simulink model "swingup_LQR"  (R2020b)
settings: Solver=VariableStepAuto  StartTime=0.0  StopTime=40  RelTol=1e-3
values from neighbouring files (symbols this model uses):
  g = 9.81    [upright_LQR.m]
  h = 0.01    [upright_LQR.m]
  Jp = mp*Lp^2/3    (= 0.000133128)    [upright_LQR.m]
  K = lqr(A, B, q_lqr, r_lqr)    [upright_LQR.m]
  ke = 0.1    [upright_LQR.m]
  kt = 0.042    [upright_LQR.m]
  l = Lp/2    (= 0.0645)    [upright_LQR.m]
  mp = 0.024    [upright_LQR.m]
  mr = 0.095    [upright_LQR.m]
  r = 0.085    [upright_LQR.m]
  Rm = 8.4    [upright_LQR.m]
  u_max = 10    [upright_LQR.m]
undefined symbols (not defined in the file or in its folder): Humusoft, MF634
libraries: simulink_extras x4, simulink x4, sldrtlib x2, eeLuenbergerObserver x1
settings Model: Creator=zhehanli  LastModifiedBy=zhehanli

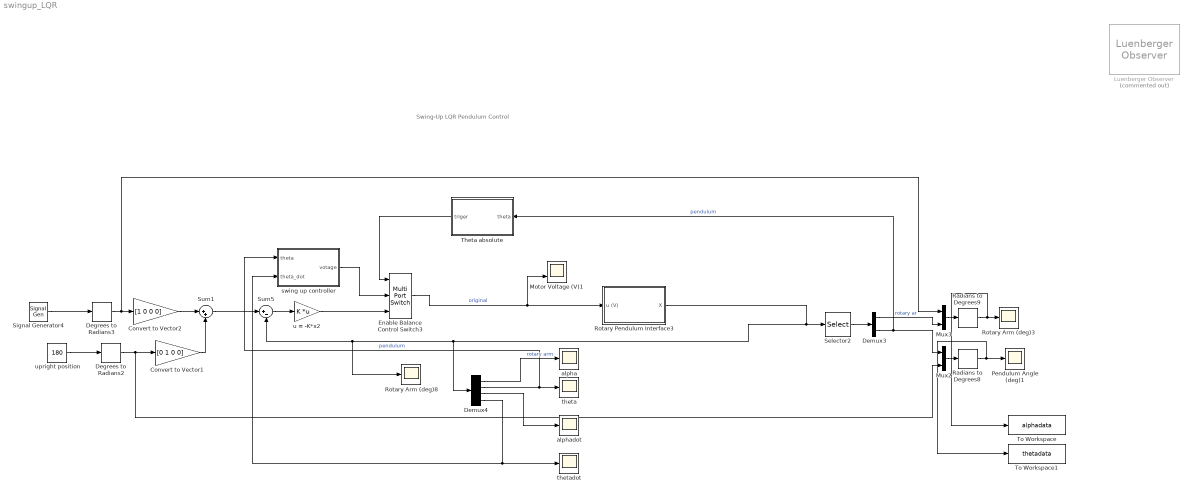
== system swingup_LQR ==
  note: Swing-Up LQR Pendulum Control
  Convert to Vector1 : Gain  Gain=[0 1 0 0]
  Convert to Vector2 : Gain  Gain=[1 0 0 0]
  Degrees to Radians2 : simulink_extras/Transformations/Degrees to Radians
  Degrees to Radians3 : simulink_extras/Transformations/Degrees to Radians
  Demux3 : Demux  Outputs=2
  Demux4 : Demux
  Enable Balance Control Switch3 : MultiPortSwitch  DataPortOrder=Zero-based contiguous  Inputs=2  zeroidx=on
  Luenberger Observer : eeLuenbergerObserver/Luenberger Observer  Commented=on  StateSpaceType=Discrete-time  Ad=1  Bd=1  Cd=1  Dd=1  A=1  B=1  C=1  D=1  ObserverDesign=Desired eigenvalues  Ld=1  DesiredEigenvalues=0  x0=0  Tsd=0.1  Ts=0.1
      settings: SourceProductBaseCode=PS
  Motor Voltage (V)1 : Scope  NumInputPorts=2
  Mux2 : Mux  Inputs=2
  Mux3 : Mux  Inputs=2
  Pendulum Angle (deg)1 : Scope
  Radians to Degrees8 : simulink_extras/Transformations/Radians to Degrees
  Radians to Degrees9 : simulink_extras/Transformations/Radians to Degrees
  Rotary Arm (deg)3 : Scope
  Rotary Arm (deg)8 : Scope
  Rotary Pendulum Interface3 : Subsystem
  Selector2 : Selector  InputPortWidth=4  IndexOptions=Index vector (dialog)  Indices=[1 2]  OutputSizes=1
  Signal Generator4 : SignalGenerator  Amplitude=20  Frequency=0.5  Units=rad/sec
  Sum1 : Sum  Inputs=|++
  Sum5 : Sum  Inputs=|+-
  Theta absolute : Subsystem
  To Workspace : ToWorkspace  VariableName=alphadata  SaveFormat=Timeseries  SampleTime=h
      settings: Decimation=2
  To Workspace1 : ToWorkspace  VariableName=thetadata  SaveFormat=Timeseries  SampleTime=h
      settings: Decimation=2
  alpha : Scope
  alphadot : Scope
  swing up controller : Subsystem
  theta : Scope
  thetadot : Scope
  u = -K*x2 : Gain  Gain=K  Multiplication=Matrix(K*u)
  upright position : Constant  Value=180  SampleTime=0
  wires:
  Sum1/1 -> Sum5/1
  Demux3/2 -> Mux2/1, Theta absolute/1(theta)  "pendulum"
  Convert to Vector1/1 -> Sum1/2
  u = -K*x2/1 -> Enable Balance Control Switch3/3
  Demux3/1 -> Mux3/2  "rotary ar"
  Radians to Degrees9/1 -> To Workspace/1, Rotary Arm (deg)3/1
  Signal Generator4/1 -> Degrees to Radians3/1
  upright position/1 -> Degrees to Radians2/1
  Demux4/1 -> alpha/1  "rotary arm"
  Convert to Vector2/1 -> Sum1/1
  Demux4/2 -> swing up controller/1(theta), theta/1  "pendulum"
  Demux4/3 -> alphadot/1
  Mux2/1 -> Radians to Degrees8/1
  Rotary Pendulum Interface3/1(X) -> Demux4/1, Rotary Arm (deg)8/1, Sum5/2, Selector2/1
  Radians to Degrees8/1 -> To Workspace1/1, Pendulum Angle (deg)1/1
  Selector2/1 -> Demux3/1
  Theta absolute/1(triger) -> Enable Balance Control Switch3/1
  Sum5/1 -> u = -K*x2/1
  Degrees to Radians2/1 -> Mux2/2, Convert to Vector1/1
  Enable Balance Control Switch3/1 -> Rotary Pendulum Interface3/1(u (V)), Motor Voltage (V)1/2  "original"
  Mux3/1 -> Radians to Degrees9/1
  Demux4/4 -> thetadot/1, swing up controller/2(theta_dot)
  Degrees to Radians3/1 -> Mux3/1, Convert to Vector2/1
  swing up controller/1(votage) -> Enable Balance Control Switch3/2

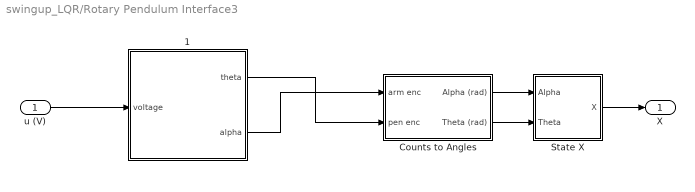
== system swingup_LQR/Rotary Pendulum Interface3 ==
  u (V) : Inport
  " 1" : Subsystem  LoadFcn=hwinit  InitFcn=hwinit  mask{h=h}
      mask prompts: h "Sampling period [s]"
      mask Display:
      | disp('Qube-Servo')
      | port_label('output',1,'theta')
      | port_label('output',2,'alpha')
      | port_label('input',1,'V')
  Counts to Angles : Subsystem
  State X : Subsystem
  X : Outport  VectorParamsAs1DForOutWhenUnconnected=off
  wires:
  u (V)/1 -> " 1"/1(voltage)
  " 1"/1(theta) -> Counts to Angles/2(pen enc)
  " 1"/2(alpha) -> Counts to Angles/1(arm enc)
  Counts to Angles/2(Theta (rad)) -> State X/2(Theta)
  Counts to Angles/1(Alpha (rad)) -> State X/1(Alpha)
  State X/1(X) -> X/1

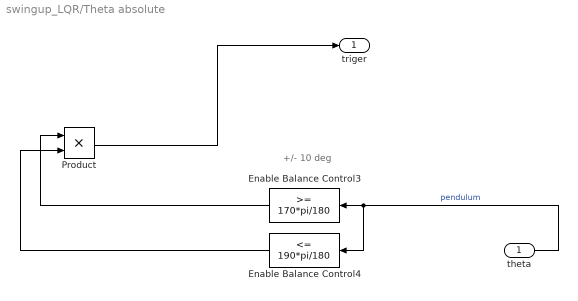
== system swingup_LQR/Theta absolute ==
  note: +/- 10 deg
  theta : Inport
  Enable Balance Control3 : simulink/Logic and Bit Operations/Compare To Constant  relop=>=  const=170*pi/180  OutDataTypeStr=uint8  ZeroCross=off
  Enable Balance Control4 : simulink/Logic and Bit Operations/Compare To Constant  relop=<=  const=190*pi/180  OutDataTypeStr=uint8  ZeroCross=off
  Product : Product
  triger : Outport  VectorParamsAs1DForOutWhenUnconnected=off
  wires:
  Enable Balance Control3/1 -> Product/1
  theta/1 -> Enable Balance Control4/1, Enable Balance Control3/1  "pendulum"
  Enable Balance Control4/1 -> Product/2
  Product/1 -> triger/1

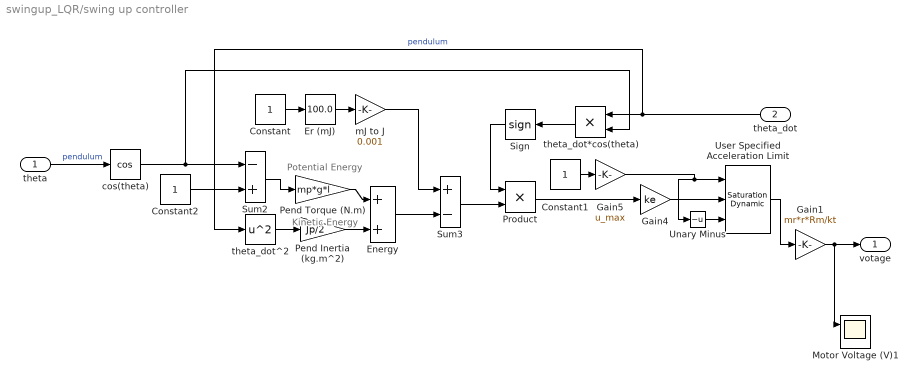
== system swingup_LQR/swing up controller ==
  note: Kinetic Energy
  note: Potential Energy
  theta : Inport
  theta_dot : Inport  Port=2
  Constant : Constant
  Constant1 : Constant
  Constant2 : Constant
  Energy : Sum  SaturateOnIntegerOverflow=on
  Er (mJ) : simulink/Math Operations/Slider Gain  gain=100.0  low=0  high=100
  Gain1 : Gain  Gain=mr*r*Rm/kt
  Gain4 : Gain  Gain=ke
  Gain5 : Gain  Gain=u_max
  Motor Voltage (V)1 : Scope  NumInputPorts=2
  Pend Inertia (kg.m^2) : Gain  Gain=Jp/2
  Pend Torque (N.m) : Gain  Gain=mp*g*l
  Product : Product  RndMeth=Zero
  Sign : Signum
  Sum2 : Sum  Inputs=-+  SaturateOnIntegerOverflow=on
  Sum3 : Sum  Inputs=+-  SaturateOnIntegerOverflow=on
  Unary Minus : UnaryMinus
  User Specified Acceleration Limit : simulink/Discontinuities/Saturation Dynamic  OutMin=-u_max  OutMax=u_max  OutDataTypeStr=Inherit: Same as second input  OutDataType=fixdt(1, 16)  OutScaling=2^-10  DoSatur=off
  cos(theta) : Trigonometry  Operator=cos
  mJ to J : Gain  Gain=0.001
  theta_dot*cos(theta) : Product  RndMeth=Zero
  theta_dot^2 : Math  Operator=square  SignedPower=on  SaturateOnIntegerOverflow=on
  votage : Outport  VectorParamsAs1DForOutWhenUnconnected=off
  wires:
  Gain5/1 -> Unary Minus/1, User Specified Acceleration Limit/1
  Constant1/1 -> Gain5/1
  Er (mJ)/1 -> mJ to J/1
  User Specified Acceleration Limit/1 -> Gain1/1
  Energy/1 -> Sum3/2
  theta_dot*cos(theta)/1 -> Sign/1
  Constant2/1 -> Sum2/2
  Sum2/1 -> Pend Torque (N.m)/1
  Pend Torque (N.m)/1 -> Energy/1
  theta_dot^2/1 -> Pend Inertia (kg.m^2)/1
  Sum3/1 -> Product/2
  Product/1 -> Gain4/1
  Gain1/1 -> Motor Voltage (V)1/1, votage/1
  Sign/1 -> Product/1
  Constant/1 -> Er (mJ)/1
  Unary Minus/1 -> User Specified Acceleration Limit/3
  Gain4/1 -> User Specified Acceleration Limit/2
  Pend Inertia (kg.m^2)/1 -> Energy/2
  mJ to J/1 -> Sum3/1
  theta/1 -> cos(theta)/1  "pendulum"
  cos(theta)/1 -> theta_dot*cos(theta)/2, Sum2/1
  theta_dot/1 -> theta_dot^2/1, theta_dot*cos(theta)/1  "pendulum"

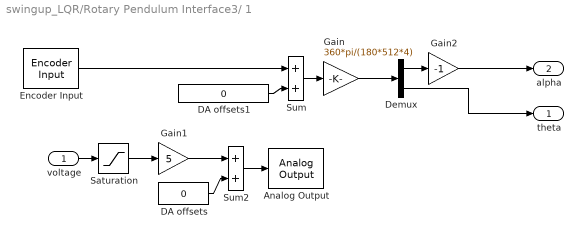
== system swingup_LQR/Rotary Pendulum Interface3/ 1 ==
  voltage : Inport
  Analog Output : sldrtlib/Analog Output  SampleTime=h  MaxMissedTicks=100  ShowMissedTicks=off  YieldWhenWaiting=off  DrvName=Humusoft/MF634  DrvAddress=4294967295  DrvOptions=0  Channels=[1]  RangeMode=2  VoltRange=1  InitialValue=0  FinalValue=0
      settings: AttributesFormatString=Humusoft\nMF634 [auto]
  DA offsets : Constant  Value=0
  DA offsets1 : Constant  Value=0  SampleTime=h
  Demux : Demux  Outputs=2
  Encoder Input : sldrtlib/Encoder Input  SampleTime=h  MaxMissedTicks=100  ShowMissedTicks=off  YieldWhenWaiting=off  DrvName=Humusoft/MF634  DrvAddress=4294967295  DrvOptions=0  Channels=[1,2]  QuadMode=3  IndexPulse=1  InputFilter=Inf  DataType=1
      settings: AttributesFormatString=Humusoft\nMF634 [auto]
  Gain : Gain  Gain=360*pi/(180*512*4)  SaturateOnIntegerOverflow=on  OutDataTypeStr=Inherit: Same as input  ParamDataTypeStr=Inherit: Same as input
  Gain1 : Gain  Gain=5  SaturateOnIntegerOverflow=on  OutDataTypeStr=Inherit: Same as input  ParamDataTypeStr=Inherit: Same as input
  Gain2 : Gain  Gain=-1  SaturateOnIntegerOverflow=on  OutDataTypeStr=Inherit: Same as input  ParamDataTypeStr=Inherit: Same as input
  Saturation : Saturate  UpperLimit=1  LowerLimit=-1
  Sum : Sum  InputSameDT=on  SaturateOnIntegerOverflow=on  OutDataTypeStr=Inherit: Same as first input
  Sum2 : Sum  InputSameDT=on  SaturateOnIntegerOverflow=on  OutDataTypeStr=Inherit: Same as first input
  theta : Outport  Tag=Cable length
  alpha : Outport  Tag=Cable length  Port=2
  wires:
  Sum/1 -> Gain/1
  DA offsets1/1 -> Sum/2
  Gain1/1 -> Sum2/1
  Sum2/1 -> Analog Output/1
  DA offsets/1 -> Sum2/2
  voltage/1 -> Saturation/1
  Encoder Input/1 -> Sum/1
  Saturation/1 -> Gain1/1
  Demux/1 -> Gain2/1
  Gain/1 -> Demux/1
  Gain2/1 -> alpha/1
  Demux/2 -> theta/1

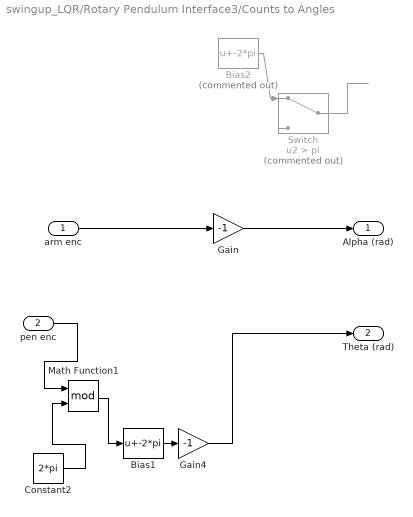
== system swingup_LQR/Rotary Pendulum Interface3/Counts to Angles ==
  arm enc : Inport
  pen enc : Inport  Port=2
  Bias1 : Bias  Bias=-2*pi
  Bias2 : Bias  Commented=on  Bias=-2*pi
  Constant2 : Constant  Value=2*pi
  Gain : Gain  Gain=-1
  Gain4 : Gain  Gain=-1
  Math Function1 : Math  Operator=mod  SignedPower=on  SaturateOnIntegerOverflow=on
  Switch : Switch  Commented=on  Criteria=u2 > Threshold  Threshold=pi
  Alpha (rad) : Outport  VectorParamsAs1DForOutWhenUnconnected=off
  Theta (rad) : Outport  Port=2  VectorParamsAs1DForOutWhenUnconnected=off
  wires:
  arm enc/1 -> Gain/1
  Gain4/1 -> Theta (rad)/1
  Math Function1/1 -> Bias1/1
  pen enc/1 -> Math Function1/1
  Constant2/1 -> Math Function1/2
  Bias1/1 -> Gain4/1
  Gain/1 -> Alpha (rad)/1
  Switch/1 -> ?
  Bias2/1 -> Switch/1
  ? -> Switch/2, Bias2/1

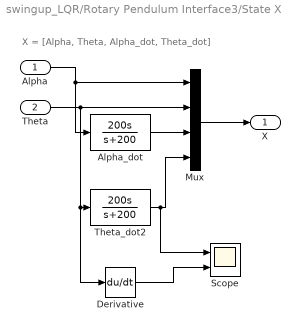
== system swingup_LQR/Rotary Pendulum Interface3/State X ==
  note: X = [Alpha, Theta, Alpha_dot, Theta_dot]
  Alpha : Inport
  Theta : Inport  Port=2
  Alpha_dot : TransferFcn  Numerator=[200 0]  Denominator=[1 200]
  Derivative : Derivative
  Mux : Mux
  Scope : Scope  NumInputPorts=2
  Theta_dot2 : TransferFcn  Numerator=[200 0]  Denominator=[1 200]
  X : Outport  VectorParamsAs1DForOutWhenUnconnected=off
  wires:
  Alpha_dot/1 -> Mux/3
  Mux/1 -> X/1
  Alpha/1 -> Mux/1, Alpha_dot/1
  Theta/1 -> Derivative/1, Theta_dot2/1, Mux/2
  Theta_dot2/1 -> Scope/1, Mux/4
  Derivative/1 -> Scope/2
